simulink model "Audio_Filter"  (R2016a)
settings: Solver=FixedStepDiscrete  SolverMode=SingleTasking  StartTime=0.0  StopTime=inf  RelTol=1e-3
undefined symbols (not defined in the file or in its folder): fdesignblkfcn, gcbh
libraries: dspindex x4, dspfdesign x2, dspsnks4 x1, dspvision x1
settings Model: Creator=Arna  LastModifiedBy=Arna
settings SolverCC: AutoInsertRateTranBlk=on
settings DataIOCC: LimitDataPoints=on  SaveOutput=off  SignalLogging=off  SaveTime=off
settings DebuggingCC: AlgebraicLoopMsg=error  SingleTaskRateTransMsg=error  AllowSymbolicDim=off
settings ConfigComp: CovModelRefEnable=Off  CovSFcnEnable=off

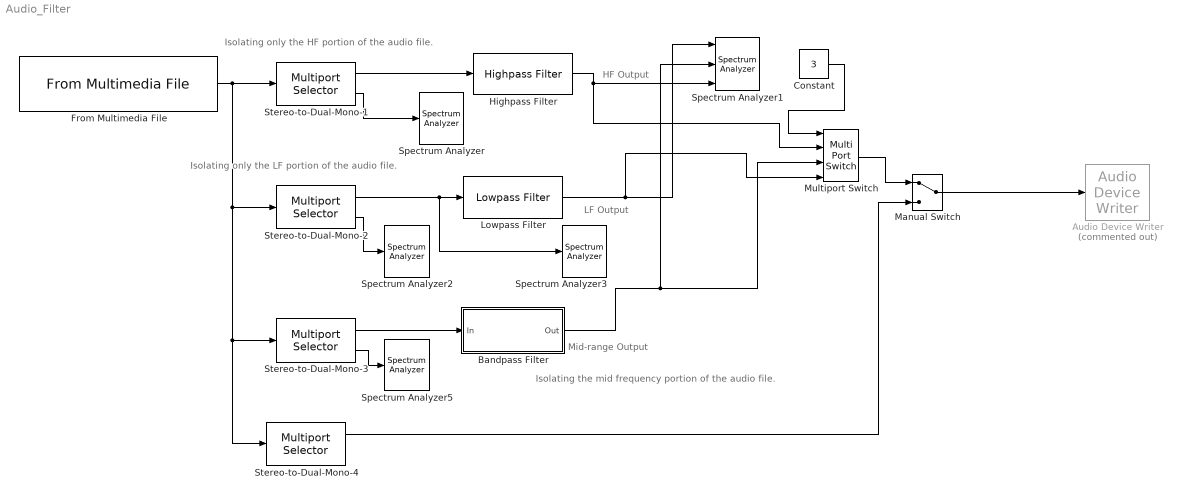
== system Audio_Filter ==
  note: Isolating the mid frequency portion of the audio file.
  note: Mid-range Output
  note: LF Output
  note: HF Output
  note: Isolating only the LF portion of the audio file.
  note: Isolating only the HF portion of the audio file.
  Audio Device Writer : dspsnks4/Audio Device Writer  Commented=on  Driver=DirectSound  Device=Default  InheritSampleRate=on  SampleRate=44100  BitDepth=16-bit integer  BufferSize=4096  NumBuffers=10  DefaultOutputChannelMapping=on  OutputChannelMapping=1:2  OutputNumUnderrunSamples=off  DriverIdx=1  DeviceWarnFlag=''
  Bandpass Filter : Subsystem  DialogController=fdesignblkfcn  InitFcn=fdesignblkfcn(gcbh, {'InitFcn'});  mask(Bandpass Filter){}
      mask help: Design a bandpass filter
      settings: CopyFcn=fdesignblkfcn(gcbh, {'CopyFcn'});
      mask Help: helpview(mapfilelocation('dsp'), 'dspbandpassfilter');
      mask Display: disp('Bandpass');
  Constant : Constant  Value=3
  From Multimedia File : dspvision/From Multimedia File  inputFilename=C:\Users\Arna\Downloads\Swell - I'm Sorry (feat. Shiloh Dynasty).mp3  loop=on  numPlays=inf  outputStreams=Audio only  videoDataType=single  audioDataType=double  inheritSampleTime=on  userDefinedSampleTime=1/30  noAudioOutput=off  isIntensityVideo=off  fourcc=RGB  colorVideoFormat=Separate color signals  outputEOF=off  dataOrg=Column-major  audioFrameSize=1024  computeAudioFrameSize=off  outSamplingMode=Sample based
  Highpass Filter : dspfdesign/Highpass Filter  FilterType=FIR  DesignForMinimumOrder=on  FilterOrder=50  StopbandFrequency=5e3  PassbandFrequency=8e3  StopbandAttenuation=80  PassbandRipple=0.1  InheritSampleRate=off  SampleRate=44100  roundingMode=Floor  coeffsDataTypeStr=fixdt(1,16)  SimulateUsing=Interpreted execution
  Lowpass Filter : dspfdesign/Lowpass Filter  FilterType=FIR  DesignForMinimumOrder=on  FilterOrder=50  PassbandFrequency=200  StopbandFrequency=2000  PassbandRipple=0.1  StopbandAttenuation=80  InheritSampleRate=off  SampleRate=44100  roundingMode=Floor  coeffsDataTypeStr=fixdt(1,16)  SimulateUsing=Interpreted execution
  Manual Switch : ManualSwitch
  Multiport Switch : MultiPortSwitch
  Spectrum Analyzer{,2..3,5} (4 alike) : SpectrumAnalyzer
  Spectrum Analyzer1 : SpectrumAnalyzer  NumInputPorts=3
  Stereo-to-Dual-Mono-1 : dspindex/Multiport Selector  rowsOrCols=Columns  idxCellArray={1,2}  idxErrMode=Clip Index
  "Stereo-to-Dual-Mono-2 " : dspindex/Multiport Selector  rowsOrCols=Columns  idxCellArray={1,2}  idxErrMode=Clip Index
  Stereo-to-Dual-Mono-3 : dspindex/Multiport Selector  rowsOrCols=Columns  idxCellArray={1,2}  idxErrMode=Clip Index
  Stereo-to-Dual-Mono-4 : dspindex/Multiport Selector  rowsOrCols=Columns  idxCellArray={1,2}  idxErrMode=Clip Index
  wires:
  Stereo-to-Dual-Mono-1/1 -> Highpass Filter/1
  Stereo-to-Dual-Mono-1/2 -> Spectrum Analyzer/1
  Highpass Filter/1 -> Multiport Switch/2, Spectrum Analyzer1/3
  From Multimedia File/1 -> Stereo-to-Dual-Mono-3/1, Stereo-to-Dual-Mono-4/1, "Stereo-to-Dual-Mono-2 "/1, Stereo-to-Dual-Mono-1/1
  "Stereo-to-Dual-Mono-2 "/1 -> Spectrum Analyzer3/1, Lowpass Filter/1
  "Stereo-to-Dual-Mono-2 "/2 -> Spectrum Analyzer2/1
  Lowpass Filter/1 -> Spectrum Analyzer1/1, Multiport Switch/4
  Manual Switch/1 -> Audio Device Writer/1
  Multiport Switch/1 -> Manual Switch/1
  Stereo-to-Dual-Mono-3/1 -> Bandpass Filter/1(In)
  Bandpass Filter/1(Out) -> Spectrum Analyzer1/2, Multiport Switch/3
  Stereo-to-Dual-Mono-3/2 -> Spectrum Analyzer5/1
  Stereo-to-Dual-Mono-4/1 -> Manual Switch/2
  Constant/1 -> Multiport Switch/1

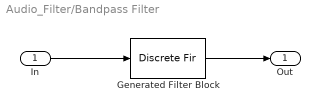
== system Audio_Filter/Bandpass Filter ==
  In : Inport
  Generated Filter Block : DiscreteFir  Tag=BlockMethodSubSystem  Coefficients=[-0.0008161542330748264 -0.0006985692233147841 -0.00066249756309064601 -0.00040609236233489959 -4.720330252651373e-05 0.00023947338913286255 0.00035375312676766283 0.00037560615364873594 0.00056073768731772331 0.0011898816100664991 0.0023391507931190738 0.0037078005010436317 0.0046483068985772634 0.0044358738110500022 0.0026741355052448327 -0.0003841598489504642 -0.0038088906588030881 -0.0063419995870890996 -0.0069879768688132712 -0.0055476267121125451 -0.0027802477969480505 -7.2345218812612587e-05 0.0012650316122166021 0.00069502300596373007 -0.0012472687304815086 -0.0032379586900965298 -0.003914768695924796 -0.0026622102531853134 1.3566365772814754e-05 0.0027674350219829428 0.0042055909960475642 0.0037287200685612305 0.0019144745505912011 0.000184859917067524 -6.6929445116742045e-05 0.00162918501246796 0.0044642610173404648 0.0067851509961277196 0.0070919792700664779 0.004998319326295398 0.0015444932787241417 -0.0013746758576043986 -0.0021593116695104264 -0.00054020857431964081 0.0021706253367004056 0.0038202115129390484 0.0027456866197325003 -0.0011140032424789446 -0.0060489918601324549 -0.0095240771035564834 -0.0097167178123090617 -0.006707710793258573 -0.0025442411082063133 -5.4646406007579876e-05 -0.001082307742329936 -0.0052234982488712943 -0.0099105974754221879 -0.011886906883266086 -0.0092362927991586474 -0.0027157255056188614 0.0045123793259248283 0.0086986344161300178 0.0078376995316109359 0.0030657646239210211 -0.0018405015428106034 -0.0026979507356235536 0.0024002811634110796 0.011624284625658241 0.020209057675851395 0.023203233251850513 0.018590971519119693 0.0088316566133009849 -0.00030844081656223189 -0.0031490960383492822 0.0022256995872438393 0.012313092232920578 0.019824312120866109 0.017926318964176156 0.0047023734036107049 -0.014961092610001121 -0.03156111602989959 -0.036381070473630574 -0.027156651721056597 -0.010523585498681116 0.0007212455235681511 -0.0053554786631157484 -0.032075850607998786 -0.070124569627813216 -0.10010549134178938 -0.10117489226829685 -0.061828442862423671 0.012642411119196187 0.10023780891495561 0.1704857358640636 0.19730654172001666 0.1704857358640636 0.10023780891495561 0.012642411119196187 -0.061828442862423671 -0.10117489226829685 -0.10010549134178938 -0.070124569627813216 -0.032075850607998786 -0.0053554786631157484 0.0007212455235681511 -0.010523585498681116 -0.027156651721056597 -0.036381070473630574 -0.03156111602989959 -0.014961092610001121 0.0047023734036107049 0.017926318964176156 0.019824312120866109 0.012313092232920578 0.0022256995872438393 -0.0031490960383492822 -0.00030844081656223189 0.0088316566133009849 0.018590971519119693 0.023203233251850513 0.020209057675851395 0.011624284625658241 0.0024002811634110796 -0.0026979507356235536 -0.0018405015428106034 0.0030657646239210211 0.0078376995316109359 0.0086986344161300178 0.0045123793259248283 -0.0027157255056188614 -0.0092362927991586474 -0.011886906883266086 -0.0099105974754221879 -0.0052234982488712943 -0.001082307742329936 -5.4646406007579876e-05 -0.0025442411082063133 -0.006707710793258573 -0.0097167178123090617 -0.0095240771035564834 -0.0060489918601324549 -0.0011140032424789446 0.0027456866197325003 0.0038202115129390484 0.0021706253367004056 -0.00054020857431964081 -0.0021593116695104264 -0.0013746758576043986 0.0015444932787241417 0.004998319326295398 0.0070919792700664779 0.0067851509961277196 0.0044642610173404648 0.00162918501246796 -6.6929445116742045e-05 0.000184859917067524 0.0019144745505912011 0.0037287200685612305 0.0042055909960475642 0.0027674350219829428 1.3566365772814754e-05 -0.0026622102531853134 -0.003914768695924796 -0.0032379586900965298 -0.0012472687304815086 0.00069502300596373007 0.0012650316122166021 -7.2345218812612587e-05 -0.0027802477969480505 -0.0055476267121125451 -0.0069879768688132712 -0.0063419995870890996 -0.0038088906588030881 -0.0003841598489504642 0.0026741355052448327 0.0044358738110500022 0.0046483068985772634 0.0037078005010436317 0.0023391507931190738 0.0011898816100664991 0.00056073768731772331 0.00037560615364873594 0.00035375312676766283 0.00023947338913286255 -4.720330252651373e-05 -0.00040609236233489959 -0.00066249756309064601 -0.0006985692233147841 -0.0008161542330748264]  InputProcessing=Columns as channels (frame based)
  Out : Outport
  wires:
  In/1 -> Generated Filter Block/1
  Generated Filter Block/1 -> Out/1
